simulink model "UR3e_collisional_model"  (R2023b)
settings: Solver=VariableStepAuto  StartTime=0.0  StopTime=60  RelTol=1e-3
model workspace: external: MATLAB File C:\Users\adoma\OneDrive - The University of Manchester\Notes\2023-24\Sem2\Individual Project\Simulation\UR3e\UR3e_DataFile.m (data not in the file)
undefined symbols (not defined in the file): simulation_parameters, smiData, X, Y, Z
libraries: sm_lib x77, nesl_utility x49, robotcorelib x1, robotmaniplib x1
(part 1 of 2)
settings Model: SimulationMode=accelerator  Creator=adoma  LastModifiedBy=user
settings ExplorerConfigSet: SimMechanicsOpenEditorOnUpdate=off

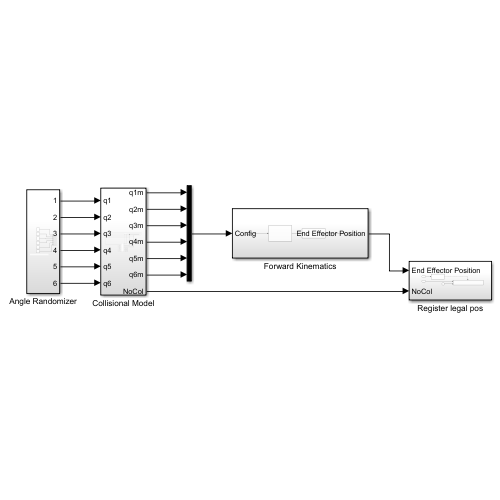
[thumbnail: Simulink's stored preview of the top-level diagram]
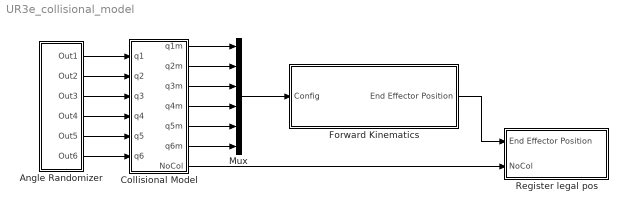
== system UR3e_collisional_model ==
  Angle Randomizer : Subsystem
  Collisional Model : Subsystem
  Forward Kinematics : Subsystem
  Mux : Mux  Inputs=6
  Register legal pos : Subsystem
  wires:
  Mux/1 -> Forward Kinematics/1(Config)
  Collisional Model/1(q1m) -> Mux/1
  Collisional Model/2(q2m) -> Mux/2
  Collisional Model/3(q3m) -> Mux/3
  Collisional Model/4(q4m) -> Mux/4
  Collisional Model/5(q5m) -> Mux/5
  Collisional Model/6(q6m) -> Mux/6
  Forward Kinematics/1(End Effector Position) -> Register legal pos/1(End Effector Position)
  Collisional Model/7(NoCol) -> Register legal pos/2(NoCol)
  Angle Randomizer/1(Out1) -> Collisional Model/1(q1)
  Angle Randomizer/2(Out2) -> Collisional Model/2(q2)
  Angle Randomizer/3(Out3) -> Collisional Model/3(q3)
  Angle Randomizer/4(Out4) -> Collisional Model/4(q4)
  Angle Randomizer/5(Out5) -> Collisional Model/5(q5)
  Angle Randomizer/6(Out6) -> Collisional Model/6(q6)

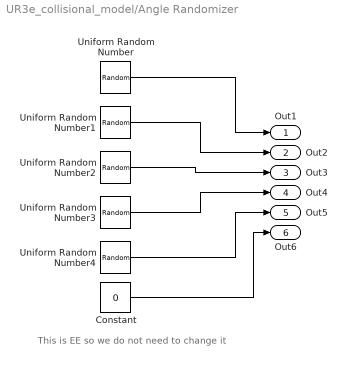
== system UR3e_collisional_model/Angle Randomizer ==
  note: This is EE so we do not need to change it
  Constant : Constant  Value=0
  Uniform Random Number : UniformRandomNumber  Minimum=-pi  Maximum=pi  SampleTime=simulation_parameters.sample_time
  Uniform Random Number1 : UniformRandomNumber  Minimum=-pi  Maximum=pi  Seed=1  SampleTime=simulation_parameters.sample_time
  Uniform Random Number2 : UniformRandomNumber  Minimum=-pi  Maximum=pi  Seed=2  SampleTime=simulation_parameters.sample_time
  Uniform Random Number3 : UniformRandomNumber  Minimum=-pi  Maximum=pi  Seed=3  SampleTime=simulation_parameters.sample_time
  Uniform Random Number4 : UniformRandomNumber  Minimum=-pi  Maximum=pi  Seed=4  SampleTime=simulation_parameters.sample_time
  Out1 : Outport
  Out2 : Outport  Port=2
  Out3 : Outport  Port=3
  Out4 : Outport  Port=4
  Out5 : Outport  Port=5
  Out6 : Outport  Port=6
  wires:
  Uniform Random Number3/1 -> Out4/1
  Uniform Random Number/1 -> Out1/1
  Uniform Random Number1/1 -> Out2/1
  Constant/1 -> Out6/1
  Uniform Random Number4/1 -> Out5/1
  Uniform Random Number2/1 -> Out3/1

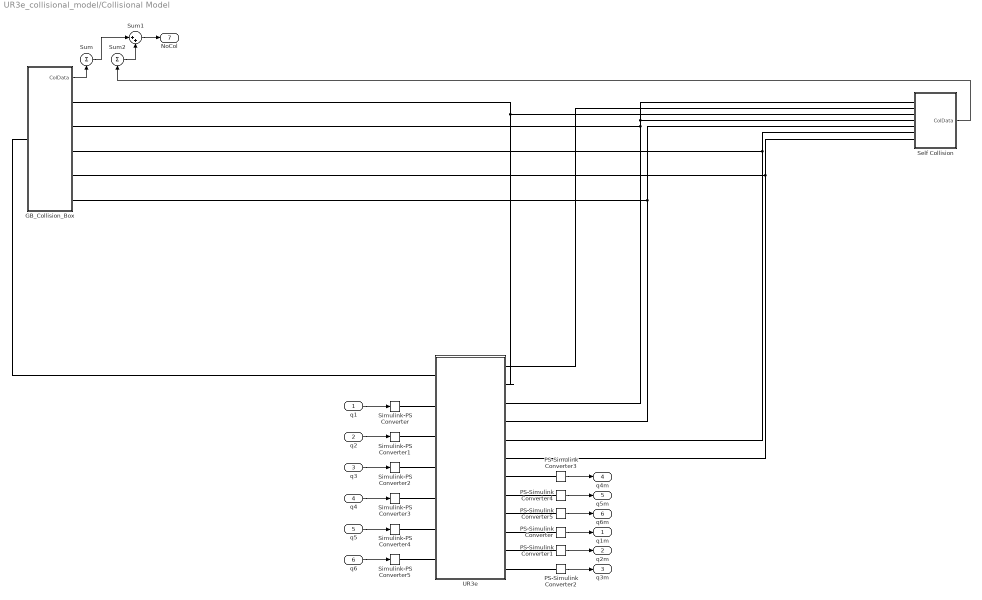
== system UR3e_collisional_model/Collisional Model ==
  q1 : Inport
  q2 : Inport  Port=2
  q3 : Inport  Port=3
  q4 : Inport  Port=4
  q5 : Inport  Port=5
  q6 : Inport  Port=6
  GB_Collision_Box : Subsystem
  PS-Simulink Converter{,1..5} (6 alike) : nesl_utility/PS-Simulink Converter  PhysicalDomain=network_engine_domain  SubClassName=ps_output  LeftPortType=input  RightPortType=output  PseudoPeriodic=off  Frequencies=[]  VectorFormat=inherit  Unit=inherit  AffineConversion=off
  Self Collision : Subsystem
  Simulink-PS Converter{,1..5} (6 alike) : nesl_utility/Simulink-PS Converter  PhysicalDomain=network_engine_domain  SubClassName=ps_input  LeftPortType=input  RightPortType=output  PseudoPeriodic=off  Frequencies=[]  NoiseDistribution=none  NoiseParameters=[]  Unit=rad  AffineConversion=off  FilteringAndDerivatives=filter  SimscapeFilterOrder=2  InputFilterTimeConstant=0.001  UdotUserProvided=0
  Sum : Sum  Inputs=|+
  Sum1 : Sum  Inputs=|++
  Sum2 : Sum  Inputs=|+
  UR3e : Subsystem
  q1m : Outport
  q2m : Outport  Port=2
  q3m : Outport  Port=3
  q4m : Outport  Port=4
  q5m : Outport  Port=5
  q6m : Outport  Port=6
  NoCol : Outport  Port=7
  wires:
  q4/1 -> Simulink-PS Converter3/1
  PS-Simulink Converter3/1 -> q4m/1
  q2/1 -> Simulink-PS Converter1/1
  PS-Simulink Converter1/1 -> q2m/1
  q5/1 -> Simulink-PS Converter4/1
  q3/1 -> Simulink-PS Converter2/1
  PS-Simulink Converter4/1 -> q5m/1
  PS-Simulink Converter5/1 -> q6m/1
  PS-Simulink Converter2/1 -> q3m/1
  q1/1 -> Simulink-PS Converter/1
  PS-Simulink Converter/1 -> q1m/1
  q6/1 -> Simulink-PS Converter5/1
  GB_Collision_Box/1(ColData) -> Sum/1
  Sum/1 -> Sum1/1
  Sum2/1 -> Sum1/2
  Sum1/1 -> NoCol/1
  Self Collision/1(ColData) -> Sum2/1
  connections:
  Self Collision/LConn7 -- UR3e/RConn6 -- GB_Collision_Box/RConn4
  GB_Collision_Box/RConn3 -- UR3e/RConn5 -- Self Collision/LConn6
  GB_Collision_Box/RConn5 -- Self Collision/LConn5 -- UR3e/RConn4
  GB_Collision_Box/LConn1 -- UR3e/LConn1
  Simulink-PS Converter/RConn1 -- UR3e/LConn2
  PS-Simulink Converter3/LConn1 -- UR3e/RConn7
  Simulink-PS Converter1/RConn1 -- UR3e/LConn3
  PS-Simulink Converter4/LConn1 -- UR3e/RConn8
  Simulink-PS Converter2/RConn1 -- UR3e/LConn4
  PS-Simulink Converter5/LConn1 -- UR3e/RConn9
  Simulink-PS Converter3/RConn1 -- UR3e/LConn5
  PS-Simulink Converter/LConn1 -- UR3e/RConn10
  Simulink-PS Converter4/RConn1 -- UR3e/LConn6
  PS-Simulink Converter1/LConn1 -- UR3e/RConn11
  Simulink-PS Converter5/RConn1 -- UR3e/LConn7
  PS-Simulink Converter2/LConn1 -- UR3e/RConn12
  UR3e/RConn2 -- GB_Collision_Box/RConn1 -- Self Collision/LConn3
  GB_Collision_Box/RConn2 -- Self Collision/LConn1 -- Self Collision/LConn4 -- UR3e/RConn3
  UR3e/RConn1 -- Self Collision/LConn2

== system UR3e_collisional_model/Forward Kinematics ==
  Config : Inport
  Coordinate Transformation Conversion : robotcorelib/Coordinate Transformation Conversion  InputRepresentation=Homogeneous Transformation  InputEulerSequence=ZYX  ShowTrVecInputPort=on  OutputRepresentation=Translation Vector  OutputEulerSequence=ZYX  ShowTrVecOutputPort=on  SimulateUsing=Interpreted execution
  Get Transform : robotmaniplib/Get Transform  RigidBodyTree=DOF6_UR3e  SourceBody=Body6  TargetBody=Base  SimulateUsing=Interpreted execution
  End Effector Position : Outport
  wires:
  Get Transform/1 -> Coordinate Transformation Conversion/1
  Coordinate Transformation Conversion/1 -> End Effector Position/1  "End Effector Position"
  Config/1 -> Get Transform/1

== system UR3e_collisional_model/Register legal pos ==
  End Effector Position : Inport
  NoCol : Inport  Port=2
  Clock : Clock
  If : If  IfExpression=u1 == 0  ShowElse=off
  Legal Position Registration : Subsystem  TreatAsAtomicUnit=on
  wires:
  NoCol/1 -> If/1
  If/1 -> Legal Position Registration/Action
  End Effector Position/1 -> Legal Position Registration/1(EE_Pos)
  Clock/1 -> Legal Position Registration/2(SimTime)

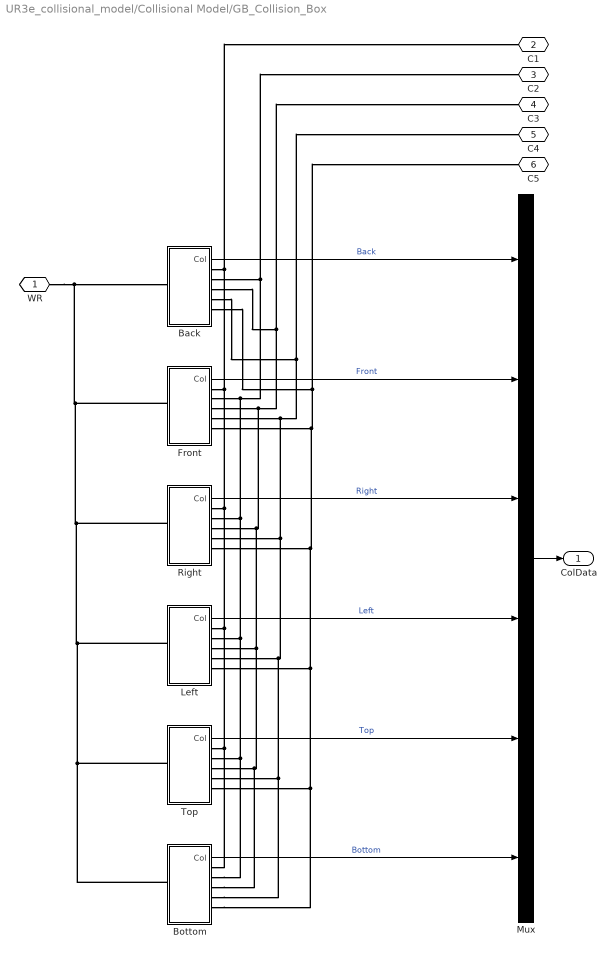
== system UR3e_collisional_model/Collisional Model/GB_Collision_Box ==
  Back : Subsystem
      settings: PortSchema="{\"entries\":[{\"content\":{\"sides\":[{\"content\":{\"connectorIds\":[\"Out1\",\"LConn1\",\"LConn2\",\"LConn3\",\"LConn4\",\"LConn5\"]},\"type\":\"ConnectorPlacement.EquallySpacedRectSide\",\"uuid\":\"f6bf8309-3a61-479f-a747-1123ec87f5cc\"},{\"content\":{\"connectorIds\":[\"RConn1\"],\"side\":\"RIGHT\"},\"type\":\"ConnectorPlacement.EquallySpacedRectSide\",\"uuid\":\"b0f1017d-061c-4274-8acc-6a947b17e7e9\"},{\"content\":{\"side\":\"TOP\"},\"type\":\"ConnectorPlacement.EquallySpacedRectSide\",\"uuid\":\"1775a24a-bc05-4d58-b171-468615c5c014\"}]},\"type\":\"ConnectorPlacement.EquallySpacedConnector\",\"uuid\":\"b2f2d87e-558d-45f7-ad7b-dc693adba59c\"}],\"packageUris\":[\"http://schema.mathworks.com/mf0/Connector/R2020b\"],\"version\":\"1.0\"}"
  Bottom : Subsystem
      settings: PortSchema="{\"entries\":[{\"content\":{\"sides\":[{\"content\":{\"connectorIds\":[\"Out1\",\"LConn1\",\"LConn2\",\"LConn3\",\"LConn4\",\"LConn5\"]},\"type\":\"ConnectorPlacement.EquallySpacedRectSide\",\"uuid\":\"f6bf8309-3a61-479f-a747-1123ec87f5cc\"},{\"content\":{\"connectorIds\":[\"RConn1\"],\"side\":\"RIGHT\"},\"type\":\"ConnectorPlacement.EquallySpacedRectSide\",\"uuid\":\"b0f1017d-061c-4274-8acc-6a947b17e7e9\"},{\"content\":{\"side\":\"TOP\"},\"type\":\"ConnectorPlacement.EquallySpacedRectSide\",\"uuid\":\"1775a24a-bc05-4d58-b171-468615c5c014\"}]},\"type\":\"ConnectorPlacement.EquallySpacedConnector\",\"uuid\":\"b2f2d87e-558d-45f7-ad7b-dc693adba59c\"}],\"packageUris\":[\"http://schema.mathworks.com/mf0/Connector/R2020b\"],\"version\":\"1.0\"}"
  Front : Subsystem
      settings: PortSchema="{\"entries\":[{\"content\":{\"sides\":[{\"content\":{\"connectorIds\":[\"Out1\",\"LConn1\",\"LConn2\",\"LConn3\",\"LConn4\",\"LConn5\"]},\"type\":\"ConnectorPlacement.EquallySpacedRectSide\",\"uuid\":\"f6bf8309-3a61-479f-a747-1123ec87f5cc\"},{\"content\":{\"connectorIds\":[\"RConn1\"],\"side\":\"RIGHT\"},\"type\":\"ConnectorPlacement.EquallySpacedRectSide\",\"uuid\":\"b0f1017d-061c-4274-8acc-6a947b17e7e9\"},{\"content\":{\"side\":\"TOP\"},\"type\":\"ConnectorPlacement.EquallySpacedRectSide\",\"uuid\":\"1775a24a-bc05-4d58-b171-468615c5c014\"}]},\"type\":\"ConnectorPlacement.EquallySpacedConnector\",\"uuid\":\"b2f2d87e-558d-45f7-ad7b-dc693adba59c\"}],\"packageUris\":[\"http://schema.mathworks.com/mf0/Connector/R2020b\"],\"version\":\"1.0\"}"
  Left : Subsystem
      settings: PortSchema="{\"entries\":[{\"content\":{\"sides\":[{\"content\":{\"connectorIds\":[\"Out1\",\"LConn1\",\"LConn2\",\"LConn3\",\"LConn4\",\"LConn5\"]},\"type\":\"ConnectorPlacement.EquallySpacedRectSide\",\"uuid\":\"f6bf8309-3a61-479f-a747-1123ec87f5cc\"},{\"content\":{\"connectorIds\":[\"RConn1\"],\"side\":\"RIGHT\"},\"type\":\"ConnectorPlacement.EquallySpacedRectSide\",\"uuid\":\"b0f1017d-061c-4274-8acc-6a947b17e7e9\"},{\"content\":{\"side\":\"TOP\"},\"type\":\"ConnectorPlacement.EquallySpacedRectSide\",\"uuid\":\"1775a24a-bc05-4d58-b171-468615c5c014\"}]},\"type\":\"ConnectorPlacement.EquallySpacedConnector\",\"uuid\":\"b2f2d87e-558d-45f7-ad7b-dc693adba59c\"}],\"packageUris\":[\"http://schema.mathworks.com/mf0/Connector/R2020b\"],\"version\":\"1.0\"}"
  Mux : Mux  Inputs=6
  Right : Subsystem
      settings: PortSchema="{\"entries\":[{\"content\":{\"sides\":[{\"content\":{\"connectorIds\":[\"Out1\",\"LConn1\",\"LConn2\",\"LConn3\",\"LConn4\",\"LConn5\"]},\"type\":\"ConnectorPlacement.EquallySpacedRectSide\",\"uuid\":\"f6bf8309-3a61-479f-a747-1123ec87f5cc\"},{\"content\":{\"connectorIds\":[\"RConn1\"],\"side\":\"RIGHT\"},\"type\":\"ConnectorPlacement.EquallySpacedRectSide\",\"uuid\":\"b0f1017d-061c-4274-8acc-6a947b17e7e9\"},{\"content\":{\"side\":\"TOP\"},\"type\":\"ConnectorPlacement.EquallySpacedRectSide\",\"uuid\":\"1775a24a-bc05-4d58-b171-468615c5c014\"}]},\"type\":\"ConnectorPlacement.EquallySpacedConnector\",\"uuid\":\"b2f2d87e-558d-45f7-ad7b-dc693adba59c\"}],\"packageUris\":[\"http://schema.mathworks.com/mf0/Connector/R2020b\"],\"version\":\"1.0\"}"
  Top : Subsystem
      settings: PortSchema="{\"entries\":[{\"content\":{\"sides\":[{\"content\":{\"connectorIds\":[\"Out1\",\"LConn1\",\"LConn2\",\"LConn3\",\"LConn4\",\"LConn5\"]},\"type\":\"ConnectorPlacement.EquallySpacedRectSide\",\"uuid\":\"f6bf8309-3a61-479f-a747-1123ec87f5cc\"},{\"content\":{\"connectorIds\":[\"RConn1\"],\"side\":\"RIGHT\"},\"type\":\"ConnectorPlacement.EquallySpacedRectSide\",\"uuid\":\"b0f1017d-061c-4274-8acc-6a947b17e7e9\"},{\"content\":{\"side\":\"TOP\"},\"type\":\"ConnectorPlacement.EquallySpacedRectSide\",\"uuid\":\"1775a24a-bc05-4d58-b171-468615c5c014\"}]},\"type\":\"ConnectorPlacement.EquallySpacedConnector\",\"uuid\":\"b2f2d87e-558d-45f7-ad7b-dc693adba59c\"}],\"packageUris\":[\"http://schema.mathworks.com/mf0/Connector/R2020b\"],\"version\":\"1.0\"}"
  WR : PMIOPort  Side=Left
  C1 : PMIOPort  Port=2  Side=Right
  C2 : PMIOPort  Port=3  Side=Right
  C3 : PMIOPort  Port=4  Side=Right
  C4 : PMIOPort  Port=5  Side=Right
  C5 : PMIOPort  Port=6  Side=Right
  ColData : Outport
  wires:
  Top/1(Col) -> Mux/5  "Top"
  Front/1(Col) -> Mux/2  "Front"
  Bottom/1(Col) -> Mux/6  "Bottom"
  Left/1(Col) -> Mux/4  "Left"
  Back/1(Col) -> Mux/1  "Back"
  Right/1(Col) -> Mux/3  "Right"
  Mux/1 -> ColData/1
  connections:
  Back/LConn4 -- Bottom/LConn4 -- Top/LConn4 -- Left/LConn4 -- Right/LConn4 -- Front/LConn4 -- C4/RConn1
  Back/LConn3 -- Bottom/LConn3 -- Top/LConn3 -- Left/LConn3 -- Right/LConn3 -- Front/LConn3 -- C3/RConn1
  Back/LConn5 -- Bottom/LConn5 -- Top/LConn5 -- Left/LConn5 -- Right/LConn5 -- Front/LConn5 -- C5/RConn1
  Back/LConn1 -- Bottom/LConn1 -- Top/LConn1 -- Left/LConn1 -- Right/LConn1 -- Front/LConn1 -- C1/RConn1
  Back/LConn2 -- Bottom/LConn2 -- Top/LConn2 -- Left/LConn2 -- Right/LConn2 -- Front/LConn2 -- C2/RConn1
  WR/RConn1 -- Bottom/RConn1 -- Top/RConn1 -- Left/RConn1 -- Right/RConn1 -- Front/RConn1 -- Back/RConn1

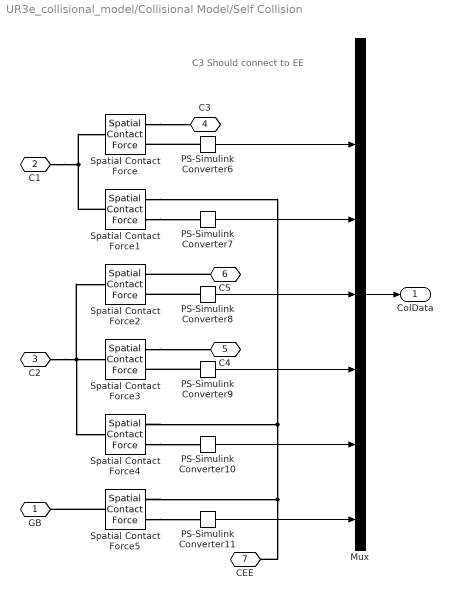
== system UR3e_collisional_model/Collisional Model/Self Collision ==
  note: C3 Should connect to EE
  Mux : Mux  Inputs=7
  PS-Simulink Converter{6..11} (6 alike) : nesl_utility/PS-Simulink Converter  PhysicalDomain=network_engine_domain  SubClassName=ps_output  LeftPortType=input  RightPortType=output  PseudoPeriodic=off  Frequencies=[]  VectorFormat=inherit  Unit=inherit  AffineConversion=off
  Spatial Contact Force{,1,3..5} (5 alike) : sm_lib/Forces and Torques/Spatial Contact Force  SenseContactBaseRotation=off  SenseContactBaseTranslation=off  CoefficientOfDynamicFriction=0.3  CoefficientOfStaticFriction=0.5  NormalDamping=1e3  NormalDampingUnits=N/(m/s)  SenseContactSignal=on  NormalStiffness=1e6  NormalStiffnessUnits=N/m  FrictionalCriticalVelocity=1e-3  FrictionalCriticalVelocityUnits=m/s  ZeroCrossDetectContactStartAndEnd=off  SenseContactFollowerRotation=off  SenseContactFollowerTranslation=off  FrictionType=SmoothStickSlip  SenseFrictionalForceMagnitude=off  SenseNormalForceMagnitude=off  NormalForceType=SmoothSpringDamper  SenseNormalVelocity=off  SensePenetrationDepth=off  SenseSeparationDistance=off  SenseTangentialVelocity=off  NormalTransitionRegionWidth=1e-4  NormalTransitionRegionWidthUnits=m
  Spatial Contact Force2 : sm_lib/Forces and Torques/Spatial Contact Force  SenseContactBaseRotation=off  SenseContactBaseTranslation=off  CoefficientOfDynamicFriction=0.3  CoefficientOfStaticFriction=0.5  NormalDamping=1e3  NormalDampingUnits=N/(m/s)  SenseContactSignal=on  NormalStiffness=1e6  NormalStiffnessUnits=N/m  FrictionalCriticalVelocity=1e-3  FrictionalCriticalVelocityUnits=m/s  ZeroCrossDetectContactStartAndEnd=on  SenseContactFollowerRotation=off  SenseContactFollowerTranslation=off  FrictionType=SmoothStickSlip  SenseFrictionalForceMagnitude=off  SenseNormalForceMagnitude=off  NormalForceType=SmoothSpringDamper  SenseNormalVelocity=off  SensePenetrationDepth=off  SenseSeparationDistance=off  SenseTangentialVelocity=off  NormalTransitionRegionWidth=1e-4  NormalTransitionRegionWidthUnits=m
  GB : PMIOPort  Side=Left
  C1 : PMIOPort  Port=2  Side=Left
  C2 : PMIOPort  Port=3  Side=Left
  C3 : PMIOPort  Port=4  Side=Left
  C4 : PMIOPort  Port=5  Side=Left
  C5 : PMIOPort  Port=6  Side=Left
  CEE : PMIOPort  Port=7  Side=Left
  ColData : Outport
  wires:
  PS-Simulink Converter10/1 -> Mux/6
  PS-Simulink Converter9/1 -> Mux/5
  PS-Simulink Converter8/1 -> Mux/4
  PS-Simulink Converter6/1 -> Mux/2
  PS-Simulink Converter7/1 -> Mux/3
  PS-Simulink Converter11/1 -> Mux/7
  Mux/1 -> ColData/1
  connections:
  C2/RConn1 -- Spatial Contact Force4/LConn1 -- Spatial Contact Force3/LConn1 -- Spatial Contact Force2/LConn1
  Spatial Contact Force3/RConn1 -- C4/RConn1
  PS-Simulink Converter6/LConn1 -- Spatial Contact Force/RConn2
  PS-Simulink Converter8/LConn1 -- Spatial Contact Force2/RConn2
  Spatial Contact Force5/RConn2 -- PS-Simulink Converter11/LConn1
  Spatial Contact Force1/RConn2 -- PS-Simulink Converter7/LConn1
  Spatial Contact Force4/RConn2 -- PS-Simulink Converter10/LConn1
  PS-Simulink Converter9/LConn1 -- Spatial Contact Force3/RConn2
  Spatial Contact Force4/RConn1 -- Spatial Contact Force1/RConn1 -- Spatial Contact Force5/RConn1 -- CEE/RConn1
  Spatial Contact Force5/LConn1 -- GB/RConn1
  C5/RConn1 -- Spatial Contact Force2/RConn1
  C1/RConn1 -- Spatial Contact Force1/LConn1 -- Spatial Contact Force/LConn1
  Spatial Contact Force/RConn1 -- C3/RConn1

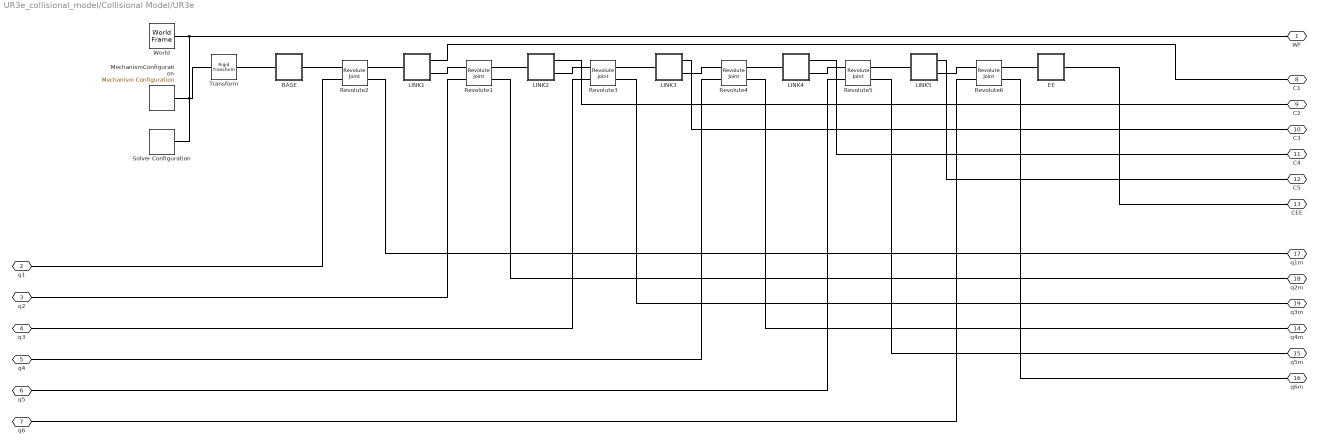
== system UR3e_collisional_model/Collisional Model/UR3e ==
  BASE : Subsystem
  EE : Subsystem
  LINK1 : Subsystem
  LINK2 : Subsystem
  LINK3 : Subsystem
  LINK4 : Subsystem
  LINK5 : Subsystem
  MechanismConfiguration : sm_lib/Utilities/Mechanism Configuration  UniformGravity=Constant  GravityVector=[0 -9.80665 0]  GravityVectorUnits=m/s^2  LinearizationDelta=0.001  JointModeTransitionNonlinearIterations=2
  Revolute{1..5} (5 alike) : sm_lib/Joints/Revolute Joint  JointMode=Normal  SenseConstraintForce=off  SenseConstraintForceX=off  SenseConstraintForceY=off  SenseConstraintForceZ=off  SenseConstraintTorque=off  SenseConstraintTorqueX=off  SenseConstraintTorqueY=off  SenseConstraintTorqueZ=off  SenseTotalForce=off  SenseTotalForceX=off  SenseTotalForceY=off  SenseTotalForceZ=off  SenseTotalTorque=off  SenseTotalTorqueX=off  SenseTotalTorqueY=off  SenseTotalTorqueZ=off  CompositeWrenchDir=FollowerOnBase  CompositeWrenchFrame=BaseFrame  EquilibriumPosition=0  EquilibriumPositionUnits=deg  SpringStiffness=0  SpringStiffnessUnits=N*m/deg  DampingCoefficient=0  DampingCoefficientUnits=N*m/(deg/s)  TorqueActuationMode=ComputedTorque  MotionActuationMode=InputMotion  SensePosition=on  SenseVelocity=off  SenseAcceleration=off  SenseTorqueForce=off  SenseLowerLimitTorqueForce=off  SenseUpperLimitTorqueForce=off  LowerLimitSpecify=on  LowerLimitBound=-360  LowerLimitBoundUnits=deg  LowerLimitStiffness=1e4  LowerLimitStiffnessUnits=N*m/deg  LowerLimitDamping=10  LowerLimitDampingUnits=N*m/(deg/s)  LowerLimitTransitionRegionWidth=0.1  LowerLimitTransitionRegionWidthUnits=deg  UpperLimitSpecify=on  UpperLimitBound=360  UpperLimitBoundUnits=deg  UpperLimitStiffness=1e4  UpperLimitStiffnessUnits=N*m/deg  UpperLimitDamping=10  UpperLimitDampingUnits=N*m/(deg/s)  UpperLimitTransitionRegionWidth=0.1  UpperLimitTransitionRegionWidthUnits=deg  PositionTargetSpecify=on  PositionTargetPriority=Low  PositionTargetValue=smiData.RevoluteJoint(3).Rz.Pos  PositionTargetValueUnits=deg  VelocityTargetSpecify=off  VelocityTargetPriority=High  VelocityTargetValue=0  VelocityTargetValueUnits=deg/s
  Revolute6 : sm_lib/Joints/Revolute Joint  JointMode=Normal  SenseConstraintForce=off  SenseConstraintForceX=off  SenseConstraintForceY=off  SenseConstraintForceZ=off  SenseConstraintTorque=off  SenseConstraintTorqueX=off  SenseConstraintTorqueY=off  SenseConstraintTorqueZ=off  SenseTotalForce=off  SenseTotalForceX=off  SenseTotalForceY=off  SenseTotalForceZ=off  SenseTotalTorque=off  SenseTotalTorqueX=off  SenseTotalTorqueY=off  SenseTotalTorqueZ=off  CompositeWrenchDir=FollowerOnBase  CompositeWrenchFrame=BaseFrame  EquilibriumPosition=0  EquilibriumPositionUnits=deg  SpringStiffness=0  SpringStiffnessUnits=N*m/deg  DampingCoefficient=0  DampingCoefficientUnits=N*m/(deg/s)  TorqueActuationMode=ComputedTorque  MotionActuationMode=InputMotion  SensePosition=on  SenseVelocity=off  SenseAcceleration=off  SenseTorqueForce=off  SenseLowerLimitTorqueForce=off  SenseUpperLimitTorqueForce=off  LowerLimitSpecify=off  LowerLimitBound=-360  LowerLimitBoundUnits=deg  LowerLimitStiffness=1e4  LowerLimitStiffnessUnits=N*m/deg  LowerLimitDamping=10  LowerLimitDampingUnits=N*m/(deg/s)  LowerLimitTransitionRegionWidth=0.1  LowerLimitTransitionRegionWidthUnits=deg  UpperLimitSpecify=off  UpperLimitBound=360  UpperLimitBoundUnits=deg  UpperLimitStiffness=1e4  UpperLimitStiffnessUnits=N*m/deg  UpperLimitDamping=10  UpperLimitDampingUnits=N*m/(deg/s)  UpperLimitTransitionRegionWidth=0.1  UpperLimitTransitionRegionWidthUnits=deg  PositionTargetSpecify=on  PositionTargetPriority=Low  PositionTargetValue=smiData.RevoluteJoint(3).Rz.Pos  PositionTargetValueUnits=deg  VelocityTargetSpecify=off  VelocityTargetPriority=High  VelocityTargetValue=0  VelocityTargetValueUnits=deg/s
  Solver Configuration : nesl_utility/Solver Configuration  PhysicalDomain=network_engine_domain  SubClassName=solver  LeftPortType=input  RightPortType=generic  Tones=[]  Harmonics=[]  SimulateNoise=off  Profile=off  UseLocalSampling=off  EnableSwitchedLinearOptims=on  FrequencyDomain=off  UseCCode=off  RelTol=0.001  AbsTol=0.001  MinStep=1e-09  ToWorkspace=off  RevertToSquareIcSolve=off  NumHomotopyIterations=100  PhasorMode=off  PhasorModeNumHarmonics=1  ConsistencySolver=NEWTON_XTOL_AFTER_FTOL  IndexReductionMethod=DerivativeReplacement  DoDC=off  ResidualTolerance=1e-09  ConsistencyTolSource=GLOBAL  ConsistencyAbsTol=0.001  ConsistencyRelTol=0.001  ConsistencyTolFactor=0.001  UseLocalSolver=off  LocalSolverChoice=NE_BACKWARD_EULER_ADVANCER  ResolveIndetEquations=on  FunctionEvalNumThread=1  LocalSolverSampleTime=0.001  DoFixedCost=off  MaxNonlinIter=3  MaxModeIter=2  ComputeImpulses=off  ImpulseIterations=2  LinearAlgebra=auto  LinearAlgebraNumThread=0  EquationFormulation=NE_TIME_EF  DelaysMemoryBudget=1024  AutomaticFiltering=on  FilteringTimeConstant=0.001  PartitionStorageMethod=AS_NEEDED  PartitionMemoryBudget=1024  PartitionMethod=ROBUST  MultibodyUseLocalSolver=off  MultibodyLocalSolverChoice=ODE1  MultibodyLocalSolverSampleTime=0.001
  Transform : sm_lib/Frames and Transforms/Rigid Transform  TranslationMethod=Cartesian  TranslationStandardOffset=0  TranslationStandardOffsetUnits=m  TranslationStandardAxis=+Z  TranslationCartesianOffset=smiData.RigidTransform(13).translation  TranslationCartesianOffsetUnits=mm  TranslationROffset=0  TranslationROffsetUnits=m  TranslationZOffset=0  TranslationZOffsetUnits=m  TranslationThetaOffset=0  TranslationThetaOffsetUnits=deg  RotationMethod=ArbitraryAxis  RotationAngleUnits=rad  RotationStandardAxis=+Z  RotationAngle=smiData.RigidTransform(13).angle  RotationArbitraryAxis=smiData.RigidTransform(13).axis  FollAlignAxisA=+X  BaseAlignAxisA=+Y  FollAlignAxisB=+Y  BaseAlignAxisB=+Z  RotationSequenceAxes=FollowerAxes  RotationSequence=XYX  RotationSequenceAngles=[0 0 0]  RotationSequenceAnglesUnits=deg  RotationMatrix=[1 0 0; 0 1 0; 0 0 1]  Quaternion=[1 0 0 0]
  World : sm_lib/Frames and Transforms/World Frame
  WF : PMIOPort  Side=Left
  q1 : PMIOPort  Port=2  Side=Left
  q2 : PMIOPort  Port=3  Side=Left
  q3 : PMIOPort  Port=4  Side=Left
  q4 : PMIOPort  Port=5  Side=Left
  q5 : PMIOPort  Port=6  Side=Left
  q6 : PMIOPort  Port=7  Side=Left
  C1 : PMIOPort  Port=8  Side=Right
  C2 : PMIOPort  Port=9  Side=Right
  C3 : PMIOPort  Port=10  Side=Right
  C4 : PMIOPort  Port=11  Side=Right
  C5 : PMIOPort  Port=12  Side=Right
  CEE : PMIOPort  Port=13  Side=Right
  q4m : PMIOPort  Port=14  Side=Right
  q5m : PMIOPort  Port=15  Side=Right
  q6m : PMIOPort  Port=16  Side=Right
  q1m : PMIOPort  Port=17  Side=Right
  q2m : PMIOPort  Port=18  Side=Right
  q3m : PMIOPort  Port=19  Side=Right
  connections:
  MechanismConfiguration/RConn1 -- Solver Configuration/RConn1 -- Transform/LConn1 -- WF/RConn1 -- World/RConn1
  Revolute4/LConn1 -- LINK3/RConn2
  Revolute5/LConn1 -- LINK4/RConn2
  Revolute4/RConn1 -- LINK4/LConn1
  Revolute3/RConn1 -- LINK3/LConn1
  LINK1/LConn1 -- Revolute2/RConn1
  Revolute6/RConn1 -- EE/LConn1
  BASE/LConn1 -- Transform/RConn1
  Revolute1/LConn1 -- LINK1/RConn2
  Revolute3/LConn1 -- LINK2/RConn2
  BASE/RConn1 -- Revolute2/LConn1
  Revolute6/LConn1 -- LINK5/RConn2
  Revolute1/RConn1 -- LINK2/LConn1
  Revolute5/RConn1 -- LINK5/LConn1
  q1/RConn1 -- Revolute2/LConn2
  q2/RConn1 -- Revolute1/LConn2
  q3/RConn1 -- Revolute3/LConn2
  q4/RConn1 -- Revolute4/LConn2
  q5/RConn1 -- Revolute5/LConn2
  q6/RConn1 -- Revolute6/LConn2
  Revolute2/RConn2 -- q1m/RConn1
  Revolute1/RConn2 -- q2m/RConn1
  Revolute3/RConn2 -- q3m/RConn1
  Revolute4/RConn2 -- q4m/RConn1
  Revolute5/RConn2 -- q5m/RConn1
  Revolute6/RConn2 -- q6m/RConn1
  LINK1/RConn1 -- C1/RConn1
  LINK2/RConn1 -- C2/RConn1
  LINK3/RConn1 -- C3/RConn1
  LINK4/RConn1 -- C4/RConn1
  LINK5/RConn1 -- C5/RConn1
  EE/RConn1 -- CEE/RConn1

== system UR3e_collisional_model/Register legal pos/Legal Position Registration ==
  EE_Pos : Inport
  SimTime : Inport  Port=2
  Action Port : ActionPort  ActionPortLabel=if(u1 == 0)
  To File : ToFile  Filename=simout.mat  MatrixName=legal_positions
  To File1 : ToFile  Commented=on  Filename=simout.mat  MatrixName=leg_time  SaveFormat=Timeseries
  wires:
  EE_Pos/1 -> To File/1
  SimTime/1 -> To File1/1

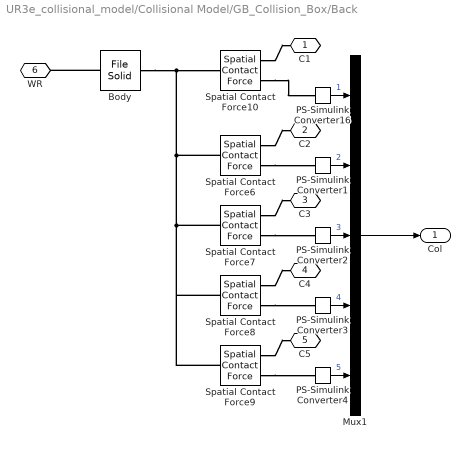
== system UR3e_collisional_model/Collisional Model/GB_Collision_Box/Back ==
  Body : sm_lib/Body Elements/File Solid  ExtGeomFileName=\UR3e_simscape_models\Glovebox_models\Back.stp  UnitType=FromFile  ExtGeomFileUnits=m  StepReaderType=HEX  ExportConvexHullGeometry=on  InertiaType=Custom  Mass=0  MassUnits=kg  CenterOfMass=[0 0 0]  CenterOfMassUnits=m  MomentsOfInertia=[1 1 1]  MomentsOfInertiaUnits=kg*m^2  ProductsOfInertia=[0 0 0]  ProductsOfInertiaUnits=kg*m^2  BasedOnType=DensityFromFile  Density=1000  DensityUnits=kg/m^3  DoExposeReferenceFrame=on  SerializedFrames=<Frames/>  GraphicType=FromGeometry  MarkerShape=Sphere  MarkerSize=10  GraphicVisPropType=SimpleVisualProperties  GraphicDiffuseColor=[1.0 1.0 1.0]  GraphicSpecularColor=[0.5 0.5 0.5 1.0]  GraphicAmbientColor=[0.15 0.15 0.15 1.0]  GraphicEmissiveColor=[0.0 0.0 0.0 1.0]  GraphicShininess=75  GraphicOpacity=0.2
  Mux1 : Mux  Inputs=5
  PS-Simulink Converter{1..4,16} (5 alike) : nesl_utility/PS-Simulink Converter  PhysicalDomain=network_engine_domain  SubClassName=ps_output  LeftPortType=input  RightPortType=output  PseudoPeriodic=off  Frequencies=[]  VectorFormat=inherit  Unit=inherit  AffineConversion=off
  Spatial Contact Force{7..10} (4 alike) : sm_lib/Forces and Torques/Spatial Contact Force  SenseContactBaseRotation=off  SenseContactBaseTranslation=off  CoefficientOfDynamicFriction=0.3  CoefficientOfStaticFriction=0.5  NormalDamping=1e3  NormalDampingUnits=N/(m/s)  SenseContactSignal=on  NormalStiffness=1e6  NormalStiffnessUnits=N/m  FrictionalCriticalVelocity=1e-3  FrictionalCriticalVelocityUnits=m/s  ZeroCrossDetectContactStartAndEnd=off  SenseContactFollowerRotation=off  SenseContactFollowerTranslation=off  FrictionType=SmoothStickSlip  SenseFrictionalForceMagnitude=off  SenseNormalForceMagnitude=off  NormalForceType=SmoothSpringDamper  SenseNormalVelocity=off  SensePenetrationDepth=off  SenseSeparationDistance=off  SenseTangentialVelocity=off  NormalTransitionRegionWidth=1e-4  NormalTransitionRegionWidthUnits=m
  Spatial Contact Force6 : sm_lib/Forces and Torques/Spatial Contact Force  SenseContactBaseRotation=off  SenseContactBaseTranslation=off  CoefficientOfDynamicFriction=0.3  CoefficientOfStaticFriction=0.5  NormalDamping=1e3  NormalDampingUnits=N/(m/s)  SenseContactSignal=on  NormalStiffness=1e6  NormalStiffnessUnits=N/m  FrictionalCriticalVelocity=1e-3  FrictionalCriticalVelocityUnits=m/s  ZeroCrossDetectContactStartAndEnd=on  SenseContactFollowerRotation=off  SenseContactFollowerTranslation=off  FrictionType=SmoothStickSlip  SenseFrictionalForceMagnitude=off  SenseNormalForceMagnitude=off  NormalForceType=SmoothSpringDamper  SenseNormalVelocity=off  SensePenetrationDepth=off  SenseSeparationDistance=off  SenseTangentialVelocity=off  NormalTransitionRegionWidth=1e-4  NormalTransitionRegionWidthUnits=m
  C1 : PMIOPort  Side=Left
  C2 : PMIOPort  Port=2  Side=Left
  C3 : PMIOPort  Port=3  Side=Left
  C4 : PMIOPort  Port=4  Side=Left
  C5 : PMIOPort  Port=5  Side=Left
  WR : PMIOPort  Port=6  Side=Right
  Col : Outport
  wires:
  PS-Simulink Converter4/1 -> Mux1/5  "5"
  PS-Simulink Converter3/1 -> Mux1/4  "4"
  PS-Simulink Converter16/1 -> Mux1/1  "1"
  PS-Simulink Converter1/1 -> Mux1/2  "2"
  PS-Simulink Converter2/1 -> Mux1/3  "3"
  Mux1/1 -> Col/1
  connections:
  Body/RConn1 -- WR/RConn1
  Body/LConn1 -- Spatial Contact Force10/LConn1 -- Spatial Contact Force9/LConn1 -- Spatial Contact Force8/LConn1 -- Spatial Contact Force7/LConn1 -- Spatial Contact Force6/LConn1
  Spatial Contact Force10/RConn1 -- C1/RConn1
  Spatial Contact Force8/RConn2 -- PS-Simulink Converter3/LConn1
  Spatial Contact Force7/RConn2 -- PS-Simulink Converter2/LConn1
  Spatial Contact Force9/RConn2 -- PS-Simulink Converter4/LConn1
  Spatial Contact Force6/RConn2 -- PS-Simulink Converter1/LConn1
  Spatial Contact Force10/RConn2 -- PS-Simulink Converter16/LConn1
  Spatial Contact Force6/RConn1 -- C2/RConn1
  Spatial Contact Force7/RConn1 -- C3/RConn1
  Spatial Contact Force8/RConn1 -- C4/RConn1
  Spatial Contact Force9/RConn1 -- C5/RConn1

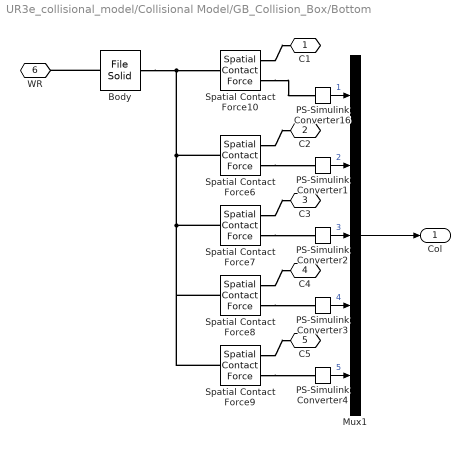
== system UR3e_collisional_model/Collisional Model/GB_Collision_Box/Bottom ==
  Body : sm_lib/Body Elements/File Solid  ExtGeomFileName=\UR3e_simscape_models\Glovebox_models\Bottom.stp  UnitType=FromFile  ExtGeomFileUnits=m  StepReaderType=HEX  ExportConvexHullGeometry=on  InertiaType=Custom  Mass=0  MassUnits=kg  CenterOfMass=[0 0 0]  CenterOfMassUnits=m  MomentsOfInertia=[1 1 1]  MomentsOfInertiaUnits=kg*m^2  ProductsOfInertia=[0 0 0]  ProductsOfInertiaUnits=kg*m^2  BasedOnType=DensityFromFile  Density=1000  DensityUnits=kg/m^3  DoExposeReferenceFrame=on  SerializedFrames=<Frames/>  GraphicType=FromGeometry  MarkerShape=Sphere  MarkerSize=10  GraphicVisPropType=SimpleVisualProperties  GraphicDiffuseColor=[1.0 1.0 1.0]  GraphicSpecularColor=[0.5 0.5 0.5 1.0]  GraphicAmbientColor=[0.15 0.15 0.15 1.0]  GraphicEmissiveColor=[0.0 0.0 0.0 1.0]  GraphicShininess=75  GraphicOpacity=0.2
  Mux1 : Mux  Inputs=5
  PS-Simulink Converter{1..4,16} (5 alike) : nesl_utility/PS-Simulink Converter  PhysicalDomain=network_engine_domain  SubClassName=ps_output  LeftPortType=input  RightPortType=output  PseudoPeriodic=off  Frequencies=[]  VectorFormat=inherit  Unit=inherit  AffineConversion=off
  Spatial Contact Force{7..10} (4 alike) : sm_lib/Forces and Torques/Spatial Contact Force  SenseContactBaseRotation=off  SenseContactBaseTranslation=off  CoefficientOfDynamicFriction=0.3  CoefficientOfStaticFriction=0.5  NormalDamping=1e3  NormalDampingUnits=N/(m/s)  SenseContactSignal=on  NormalStiffness=1e6  NormalStiffnessUnits=N/m  FrictionalCriticalVelocity=1e-3  FrictionalCriticalVelocityUnits=m/s  ZeroCrossDetectContactStartAndEnd=off  SenseContactFollowerRotation=off  SenseContactFollowerTranslation=off  FrictionType=SmoothStickSlip  SenseFrictionalForceMagnitude=off  SenseNormalForceMagnitude=off  NormalForceType=SmoothSpringDamper  SenseNormalVelocity=off  SensePenetrationDepth=off  SenseSeparationDistance=off  SenseTangentialVelocity=off  NormalTransitionRegionWidth=1e-4  NormalTransitionRegionWidthUnits=m
  Spatial Contact Force6 : sm_lib/Forces and Torques/Spatial Contact Force  SenseContactBaseRotation=off  SenseContactBaseTranslation=off  CoefficientOfDynamicFriction=0.3  CoefficientOfStaticFriction=0.5  NormalDamping=1e3  NormalDampingUnits=N/(m/s)  SenseContactSignal=on  NormalStiffness=1e6  NormalStiffnessUnits=N/m  FrictionalCriticalVelocity=1e-3  FrictionalCriticalVelocityUnits=m/s  ZeroCrossDetectContactStartAndEnd=on  SenseContactFollowerRotation=off  SenseContactFollowerTranslation=off  FrictionType=SmoothStickSlip  SenseFrictionalForceMagnitude=off  SenseNormalForceMagnitude=off  NormalForceType=SmoothSpringDamper  SenseNormalVelocity=off  SensePenetrationDepth=off  SenseSeparationDistance=off  SenseTangentialVelocity=off  NormalTransitionRegionWidth=1e-4  NormalTransitionRegionWidthUnits=m
  C1 : PMIOPort  Side=Left
  C2 : PMIOPort  Port=2  Side=Left
  C3 : PMIOPort  Port=3  Side=Left
  C4 : PMIOPort  Port=4  Side=Left
  C5 : PMIOPort  Port=5  Side=Left
  WR : PMIOPort  Port=6  Side=Right
  Col : Outport
  wires:
  PS-Simulink Converter4/1 -> Mux1/5  "5"
  PS-Simulink Converter3/1 -> Mux1/4  "4"
  PS-Simulink Converter16/1 -> Mux1/1  "1"
  PS-Simulink Converter1/1 -> Mux1/2  "2"
  PS-Simulink Converter2/1 -> Mux1/3  "3"
  Mux1/1 -> Col/1
  connections:
  Body/RConn1 -- WR/RConn1
  Body/LConn1 -- Spatial Contact Force9/LConn1 -- Spatial Contact Force8/LConn1 -- Spatial Contact Force7/LConn1 -- Spatial Contact Force6/LConn1 -- Spatial Contact Force10/LConn1
  Spatial Contact Force10/RConn1 -- C1/RConn1
  Spatial Contact Force8/RConn2 -- PS-Simulink Converter3/LConn1
  Spatial Contact Force7/RConn2 -- PS-Simulink Converter2/LConn1
  Spatial Contact Force9/RConn2 -- PS-Simulink Converter4/LConn1
  Spatial Contact Force6/RConn2 -- PS-Simulink Converter1/LConn1
  Spatial Contact Force10/RConn2 -- PS-Simulink Converter16/LConn1
  Spatial Contact Force6/RConn1 -- C2/RConn1
  Spatial Contact Force7/RConn1 -- C3/RConn1
  Spatial Contact Force8/RConn1 -- C4/RConn1
  Spatial Contact Force9/RConn1 -- C5/RConn1

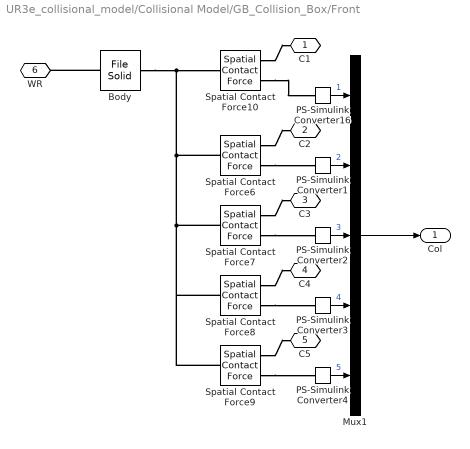
== system UR3e_collisional_model/Collisional Model/GB_Collision_Box/Front ==
  Body : sm_lib/Body Elements/File Solid  ExtGeomFileName=\UR3e_simscape_models\Glovebox_models\Front.stp  UnitType=FromFile  ExtGeomFileUnits=m  StepReaderType=HEX  ExportConvexHullGeometry=on  InertiaType=Custom  Mass=0  MassUnits=kg  CenterOfMass=[0 0 0]  CenterOfMassUnits=m  MomentsOfInertia=[1 1 1]  MomentsOfInertiaUnits=kg*m^2  ProductsOfInertia=[0 0 0]  ProductsOfInertiaUnits=kg*m^2  BasedOnType=DensityFromFile  Density=1000  DensityUnits=kg/m^3  DoExposeReferenceFrame=on  SerializedFrames=<Frames/>  GraphicType=FromGeometry  MarkerShape=Sphere  MarkerSize=10  GraphicVisPropType=SimpleVisualProperties  GraphicDiffuseColor=[1.0 1.0 1.0]  GraphicSpecularColor=[0.5 0.5 0.5 1.0]  GraphicAmbientColor=[0.15 0.15 0.15 1.0]  GraphicEmissiveColor=[0.0 0.0 0.0 1.0]  GraphicShininess=75  GraphicOpacity=0.2
  Mux1 : Mux  Inputs=5
  PS-Simulink Converter{1..4,16} (5 alike) : nesl_utility/PS-Simulink Converter  PhysicalDomain=network_engine_domain  SubClassName=ps_output  LeftPortType=input  RightPortType=output  PseudoPeriodic=off  Frequencies=[]  VectorFormat=inherit  Unit=inherit  AffineConversion=off
  Spatial Contact Force{7..10} (4 alike) : sm_lib/Forces and Torques/Spatial Contact Force  SenseContactBaseRotation=off  SenseContactBaseTranslation=off  CoefficientOfDynamicFriction=0.3  CoefficientOfStaticFriction=0.5  NormalDamping=1e3  NormalDampingUnits=N/(m/s)  SenseContactSignal=on  NormalStiffness=1e6  NormalStiffnessUnits=N/m  FrictionalCriticalVelocity=1e-3  FrictionalCriticalVelocityUnits=m/s  ZeroCrossDetectContactStartAndEnd=off  SenseContactFollowerRotation=off  SenseContactFollowerTranslation=off  FrictionType=SmoothStickSlip  SenseFrictionalForceMagnitude=off  SenseNormalForceMagnitude=off  NormalForceType=SmoothSpringDamper  SenseNormalVelocity=off  SensePenetrationDepth=off  SenseSeparationDistance=off  SenseTangentialVelocity=off  NormalTransitionRegionWidth=1e-4  NormalTransitionRegionWidthUnits=m
  Spatial Contact Force6 : sm_lib/Forces and Torques/Spatial Contact Force  SenseContactBaseRotation=off  SenseContactBaseTranslation=off  CoefficientOfDynamicFriction=0.3  CoefficientOfStaticFriction=0.5  NormalDamping=1e3  NormalDampingUnits=N/(m/s)  SenseContactSignal=on  NormalStiffness=1e6  NormalStiffnessUnits=N/m  FrictionalCriticalVelocity=1e-3  FrictionalCriticalVelocityUnits=m/s  ZeroCrossDetectContactStartAndEnd=on  SenseContactFollowerRotation=off  SenseContactFollowerTranslation=off  FrictionType=SmoothStickSlip  SenseFrictionalForceMagnitude=off  SenseNormalForceMagnitude=off  NormalForceType=SmoothSpringDamper  SenseNormalVelocity=off  SensePenetrationDepth=off  SenseSeparationDistance=off  SenseTangentialVelocity=off  NormalTransitionRegionWidth=1e-4  NormalTransitionRegionWidthUnits=m
  C1 : PMIOPort  Side=Left
  C2 : PMIOPort  Port=2  Side=Left
  C3 : PMIOPort  Port=3  Side=Left
  C4 : PMIOPort  Port=4  Side=Left
  C5 : PMIOPort  Port=5  Side=Left
  WR : PMIOPort  Port=6  Side=Right
  Col : Outport
  wires:
  PS-Simulink Converter4/1 -> Mux1/5  "5"
  PS-Simulink Converter3/1 -> Mux1/4  "4"
  PS-Simulink Converter16/1 -> Mux1/1  "1"
  PS-Simulink Converter1/1 -> Mux1/2  "2"
  PS-Simulink Converter2/1 -> Mux1/3  "3"
  Mux1/1 -> Col/1
  connections:
  Body/RConn1 -- WR/RConn1
  Body/LConn1 -- Spatial Contact Force10/LConn1 -- Spatial Contact Force9/LConn1 -- Spatial Contact Force8/LConn1 -- Spatial Contact Force7/LConn1 -- Spatial Contact Force6/LConn1
  Spatial Contact Force10/RConn1 -- C1/RConn1
  Spatial Contact Force8/RConn2 -- PS-Simulink Converter3/LConn1
  Spatial Contact Force7/RConn2 -- PS-Simulink Converter2/LConn1
  Spatial Contact Force9/RConn2 -- PS-Simulink Converter4/LConn1
  Spatial Contact Force6/RConn2 -- PS-Simulink Converter1/LConn1
  Spatial Contact Force10/RConn2 -- PS-Simulink Converter16/LConn1
  Spatial Contact Force6/RConn1 -- C2/RConn1
  Spatial Contact Force7/RConn1 -- C3/RConn1
  Spatial Contact Force8/RConn1 -- C4/RConn1
  Spatial Contact Force9/RConn1 -- C5/RConn1

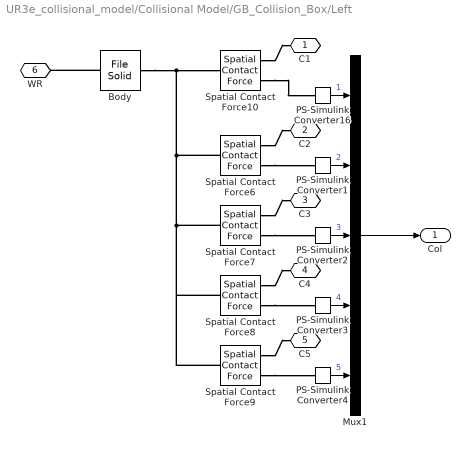
== system UR3e_collisional_model/Collisional Model/GB_Collision_Box/Left ==
  Body : sm_lib/Body Elements/File Solid  ExtGeomFileName=\UR3e_simscape_models\Glovebox_models\Left.stp  UnitType=FromFile  ExtGeomFileUnits=m  StepReaderType=HEX  ExportConvexHullGeometry=on  InertiaType=Custom  Mass=0  MassUnits=kg  CenterOfMass=[0 0 0]  CenterOfMassUnits=m  MomentsOfInertia=[1 1 1]  MomentsOfInertiaUnits=kg*m^2  ProductsOfInertia=[0 0 0]  ProductsOfInertiaUnits=kg*m^2  BasedOnType=DensityFromFile  Density=1000  DensityUnits=kg/m^3  DoExposeReferenceFrame=on  SerializedFrames=<Frames/>  GraphicType=FromGeometry  MarkerShape=Sphere  MarkerSize=10  GraphicVisPropType=SimpleVisualProperties  GraphicDiffuseColor=[1.0 1.0 1.0]  GraphicSpecularColor=[0.5 0.5 0.5 1.0]  GraphicAmbientColor=[0.15 0.15 0.15 1.0]  GraphicEmissiveColor=[0.0 0.0 0.0 1.0]  GraphicShininess=75  GraphicOpacity=0.2
  Mux1 : Mux  Inputs=5
  PS-Simulink Converter{1..4,16} (5 alike) : nesl_utility/PS-Simulink Converter  PhysicalDomain=network_engine_domain  SubClassName=ps_output  LeftPortType=input  RightPortType=output  PseudoPeriodic=off  Frequencies=[]  VectorFormat=inherit  Unit=inherit  AffineConversion=off
  Spatial Contact Force{7..10} (4 alike) : sm_lib/Forces and Torques/Spatial Contact Force  SenseContactBaseRotation=off  SenseContactBaseTranslation=off  CoefficientOfDynamicFriction=0.3  CoefficientOfStaticFriction=0.5  NormalDamping=1e3  NormalDampingUnits=N/(m/s)  SenseContactSignal=on  NormalStiffness=1e6  NormalStiffnessUnits=N/m  FrictionalCriticalVelocity=1e-3  FrictionalCriticalVelocityUnits=m/s  ZeroCrossDetectContactStartAndEnd=off  SenseContactFollowerRotation=off  SenseContactFollowerTranslation=off  FrictionType=SmoothStickSlip  SenseFrictionalForceMagnitude=off  SenseNormalForceMagnitude=off  NormalForceType=SmoothSpringDamper  SenseNormalVelocity=off  SensePenetrationDepth=off  SenseSeparationDistance=off  SenseTangentialVelocity=off  NormalTransitionRegionWidth=1e-4  NormalTransitionRegionWidthUnits=m
  Spatial Contact Force6 : sm_lib/Forces and Torques/Spatial Contact Force  SenseContactBaseRotation=off  SenseContactBaseTranslation=off  CoefficientOfDynamicFriction=0.3  CoefficientOfStaticFriction=0.5  NormalDamping=1e3  NormalDampingUnits=N/(m/s)  SenseContactSignal=on  NormalStiffness=1e6  NormalStiffnessUnits=N/m  FrictionalCriticalVelocity=1e-3  FrictionalCriticalVelocityUnits=m/s  ZeroCrossDetectContactStartAndEnd=on  SenseContactFollowerRotation=off  SenseContactFollowerTranslation=off  FrictionType=SmoothStickSlip  SenseFrictionalForceMagnitude=off  SenseNormalForceMagnitude=off  NormalForceType=SmoothSpringDamper  SenseNormalVelocity=off  SensePenetrationDepth=off  SenseSeparationDistance=off  SenseTangentialVelocity=off  NormalTransitionRegionWidth=1e-4  NormalTransitionRegionWidthUnits=m
  C1 : PMIOPort  Side=Left
  C2 : PMIOPort  Port=2  Side=Left
  C3 : PMIOPort  Port=3  Side=Left
  C4 : PMIOPort  Port=4  Side=Left
  C5 : PMIOPort  Port=5  Side=Left
  WR : PMIOPort  Port=6  Side=Right
  Col : Outport
  wires:
  PS-Simulink Converter4/1 -> Mux1/5  "5"
  PS-Simulink Converter3/1 -> Mux1/4  "4"
  PS-Simulink Converter16/1 -> Mux1/1  "1"
  PS-Simulink Converter1/1 -> Mux1/2  "2"
  PS-Simulink Converter2/1 -> Mux1/3  "3"
  Mux1/1 -> Col/1
  connections:
  Body/RConn1 -- WR/RConn1
  Body/LConn1 -- Spatial Contact Force10/LConn1 -- Spatial Contact Force9/LConn1 -- Spatial Contact Force8/LConn1 -- Spatial Contact Force7/LConn1 -- Spatial Contact Force6/LConn1
  Spatial Contact Force10/RConn1 -- C1/RConn1
  Spatial Contact Force8/RConn2 -- PS-Simulink Converter3/LConn1
  Spatial Contact Force7/RConn2 -- PS-Simulink Converter2/LConn1
  Spatial Contact Force9/RConn2 -- PS-Simulink Converter4/LConn1
  Spatial Contact Force6/RConn2 -- PS-Simulink Converter1/LConn1
  Spatial Contact Force10/RConn2 -- PS-Simulink Converter16/LConn1
  Spatial Contact Force6/RConn1 -- C2/RConn1
  Spatial Contact Force7/RConn1 -- C3/RConn1
  Spatial Contact Force8/RConn1 -- C4/RConn1
  Spatial Contact Force9/RConn1 -- C5/RConn1

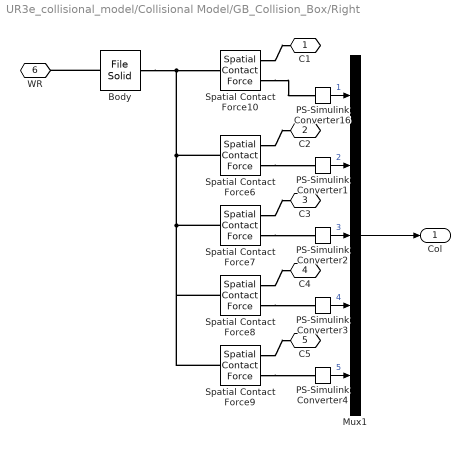
== system UR3e_collisional_model/Collisional Model/GB_Collision_Box/Right ==
  Body : sm_lib/Body Elements/File Solid  ExtGeomFileName=\UR3e_simscape_models\Glovebox_models\Right.stp  UnitType=FromFile  ExtGeomFileUnits=m  StepReaderType=HEX  ExportConvexHullGeometry=on  InertiaType=Custom  Mass=0  MassUnits=kg  CenterOfMass=[0 0 0]  CenterOfMassUnits=m  MomentsOfInertia=[1 1 1]  MomentsOfInertiaUnits=kg*m^2  ProductsOfInertia=[0 0 0]  ProductsOfInertiaUnits=kg*m^2  BasedOnType=DensityFromFile  Density=1000  DensityUnits=kg/m^3  DoExposeReferenceFrame=on  SerializedFrames=<Frames/>  GraphicType=FromGeometry  MarkerShape=Sphere  MarkerSize=10  GraphicVisPropType=SimpleVisualProperties  GraphicDiffuseColor=[1.0 1.0 1.0]  GraphicSpecularColor=[0.5 0.5 0.5 1.0]  GraphicAmbientColor=[0.15 0.15 0.15 1.0]  GraphicEmissiveColor=[0.0 0.0 0.0 1.0]  GraphicShininess=75  GraphicOpacity=0.2
  Mux1 : Mux  Inputs=5
  PS-Simulink Converter{1..4,16} (5 alike) : nesl_utility/PS-Simulink Converter  PhysicalDomain=network_engine_domain  SubClassName=ps_output  LeftPortType=input  RightPortType=output  PseudoPeriodic=off  Frequencies=[]  VectorFormat=inherit  Unit=inherit  AffineConversion=off
  Spatial Contact Force{7..10} (4 alike) : sm_lib/Forces and Torques/Spatial Contact Force  SenseContactBaseRotation=off  SenseContactBaseTranslation=off  CoefficientOfDynamicFriction=0.3  CoefficientOfStaticFriction=0.5  NormalDamping=1e3  NormalDampingUnits=N/(m/s)  SenseContactSignal=on  NormalStiffness=1e6  NormalStiffnessUnits=N/m  FrictionalCriticalVelocity=1e-3  FrictionalCriticalVelocityUnits=m/s  ZeroCrossDetectContactStartAndEnd=off  SenseContactFollowerRotation=off  SenseContactFollowerTranslation=off  FrictionType=SmoothStickSlip  SenseFrictionalForceMagnitude=off  SenseNormalForceMagnitude=off  NormalForceType=SmoothSpringDamper  SenseNormalVelocity=off  SensePenetrationDepth=off  SenseSeparationDistance=off  SenseTangentialVelocity=off  NormalTransitionRegionWidth=1e-4  NormalTransitionRegionWidthUnits=m
  Spatial Contact Force6 : sm_lib/Forces and Torques/Spatial Contact Force  SenseContactBaseRotation=off  SenseContactBaseTranslation=off  CoefficientOfDynamicFriction=0.3  CoefficientOfStaticFriction=0.5  NormalDamping=1e3  NormalDampingUnits=N/(m/s)  SenseContactSignal=on  NormalStiffness=1e6  NormalStiffnessUnits=N/m  FrictionalCriticalVelocity=1e-3  FrictionalCriticalVelocityUnits=m/s  ZeroCrossDetectContactStartAndEnd=on  SenseContactFollowerRotation=off  SenseContactFollowerTranslation=off  FrictionType=SmoothStickSlip  SenseFrictionalForceMagnitude=off  SenseNormalForceMagnitude=off  NormalForceType=SmoothSpringDamper  SenseNormalVelocity=off  SensePenetrationDepth=off  SenseSeparationDistance=off  SenseTangentialVelocity=off  NormalTransitionRegionWidth=1e-4  NormalTransitionRegionWidthUnits=m
  C1 : PMIOPort  Side=Left
  C2 : PMIOPort  Port=2  Side=Left
  C3 : PMIOPort  Port=3  Side=Left
  C4 : PMIOPort  Port=4  Side=Left
  C5 : PMIOPort  Port=5  Side=Left
  WR : PMIOPort  Port=6  Side=Right
  Col : Outport
  wires:
  PS-Simulink Converter4/1 -> Mux1/5  "5"
  PS-Simulink Converter3/1 -> Mux1/4  "4"
  PS-Simulink Converter16/1 -> Mux1/1  "1"
  PS-Simulink Converter1/1 -> Mux1/2  "2"
  PS-Simulink Converter2/1 -> Mux1/3  "3"
  Mux1/1 -> Col/1
  connections:
  Body/RConn1 -- WR/RConn1
  Body/LConn1 -- Spatial Contact Force10/LConn1 -- Spatial Contact Force9/LConn1 -- Spatial Contact Force8/LConn1 -- Spatial Contact Force7/LConn1 -- Spatial Contact Force6/LConn1
  Spatial Contact Force10/RConn1 -- C1/RConn1
  Spatial Contact Force8/RConn2 -- PS-Simulink Converter3/LConn1
  Spatial Contact Force7/RConn2 -- PS-Simulink Converter2/LConn1
  Spatial Contact Force9/RConn2 -- PS-Simulink Converter4/LConn1
  Spatial Contact Force6/RConn2 -- PS-Simulink Converter1/LConn1
  Spatial Contact Force10/RConn2 -- PS-Simulink Converter16/LConn1
  Spatial Contact Force6/RConn1 -- C2/RConn1
  Spatial Contact Force7/RConn1 -- C3/RConn1
  Spatial Contact Force8/RConn1 -- C4/RConn1
  Spatial Contact Force9/RConn1 -- C5/RConn1

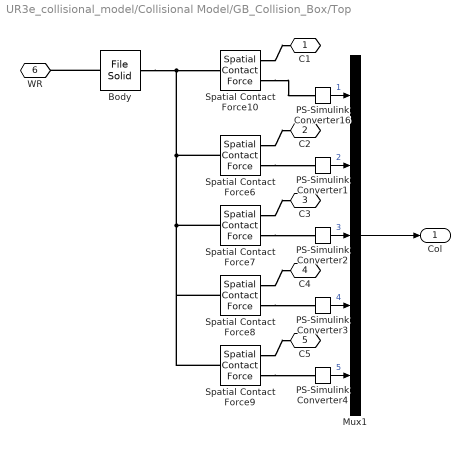
== system UR3e_collisional_model/Collisional Model/GB_Collision_Box/Top ==
  Body : sm_lib/Body Elements/File Solid  ExtGeomFileName=\UR3e_simscape_models\Glovebox_models\Top.stp  UnitType=FromFile  ExtGeomFileUnits=m  StepReaderType=HEX  ExportConvexHullGeometry=on  InertiaType=Custom  Mass=0  MassUnits=kg  CenterOfMass=[0 0 0]  CenterOfMassUnits=m  MomentsOfInertia=[1 1 1]  MomentsOfInertiaUnits=kg*m^2  ProductsOfInertia=[0 0 0]  ProductsOfInertiaUnits=kg*m^2  BasedOnType=DensityFromFile  Density=1000  DensityUnits=kg/m^3  DoExposeReferenceFrame=on  SerializedFrames=<Frames/>  GraphicType=FromGeometry  MarkerShape=Sphere  MarkerSize=10  GraphicVisPropType=SimpleVisualProperties  GraphicDiffuseColor=[1.0 1.0 1.0]  GraphicSpecularColor=[0.5 0.5 0.5 1.0]  GraphicAmbientColor=[0.15 0.15 0.15 1.0]  GraphicEmissiveColor=[0.0 0.0 0.0 1.0]  GraphicShininess=75  GraphicOpacity=0.2
  Mux1 : Mux  Inputs=5
  PS-Simulink Converter{1..4,16} (5 alike) : nesl_utility/PS-Simulink Converter  PhysicalDomain=network_engine_domain  SubClassName=ps_output  LeftPortType=input  RightPortType=output  PseudoPeriodic=off  Frequencies=[]  VectorFormat=inherit  Unit=inherit  AffineConversion=off
  Spatial Contact Force{7..10} (4 alike) : sm_lib/Forces and Torques/Spatial Contact Force  SenseContactBaseRotation=off  SenseContactBaseTranslation=off  CoefficientOfDynamicFriction=0.3  CoefficientOfStaticFriction=0.5  NormalDamping=1e3  NormalDampingUnits=N/(m/s)  SenseContactSignal=on  NormalStiffness=1e6  NormalStiffnessUnits=N/m  FrictionalCriticalVelocity=1e-3  FrictionalCriticalVelocityUnits=m/s  ZeroCrossDetectContactStartAndEnd=off  SenseContactFollowerRotation=off  SenseContactFollowerTranslation=off  FrictionType=SmoothStickSlip  SenseFrictionalForceMagnitude=off  SenseNormalForceMagnitude=off  NormalForceType=SmoothSpringDamper  SenseNormalVelocity=off  SensePenetrationDepth=off  SenseSeparationDistance=off  SenseTangentialVelocity=off  NormalTransitionRegionWidth=1e-4  NormalTransitionRegionWidthUnits=m
  Spatial Contact Force6 : sm_lib/Forces and Torques/Spatial Contact Force  SenseContactBaseRotation=off  SenseContactBaseTranslation=off  CoefficientOfDynamicFriction=0.3  CoefficientOfStaticFriction=0.5  NormalDamping=1e3  NormalDampingUnits=N/(m/s)  SenseContactSignal=on  NormalStiffness=1e6  NormalStiffnessUnits=N/m  FrictionalCriticalVelocity=1e-3  FrictionalCriticalVelocityUnits=m/s  ZeroCrossDetectContactStartAndEnd=on  SenseContactFollowerRotation=off  SenseContactFollowerTranslation=off  FrictionType=SmoothStickSlip  SenseFrictionalForceMagnitude=off  SenseNormalForceMagnitude=off  NormalForceType=SmoothSpringDamper  SenseNormalVelocity=off  SensePenetrationDepth=off  SenseSeparationDistance=off  SenseTangentialVelocity=off  NormalTransitionRegionWidth=1e-4  NormalTransitionRegionWidthUnits=m
  C1 : PMIOPort  Side=Left
  C2 : PMIOPort  Port=2  Side=Left
  C3 : PMIOPort  Port=3  Side=Left
  C4 : PMIOPort  Port=4  Side=Left
  C5 : PMIOPort  Port=5  Side=Left
  WR : PMIOPort  Port=6  Side=Right
  Col : Outport
  wires:
  PS-Simulink Converter4/1 -> Mux1/5  "5"
  PS-Simulink Converter3/1 -> Mux1/4  "4"
  PS-Simulink Converter16/1 -> Mux1/1  "1"
  PS-Simulink Converter1/1 -> Mux1/2  "2"
  PS-Simulink Converter2/1 -> Mux1/3  "3"
  Mux1/1 -> Col/1
  connections:
  Body/RConn1 -- WR/RConn1
  Body/LConn1 -- Spatial Contact Force10/LConn1 -- Spatial Contact Force9/LConn1 -- Spatial Contact Force8/LConn1 -- Spatial Contact Force7/LConn1 -- Spatial Contact Force6/LConn1
  Spatial Contact Force10/RConn1 -- C1/RConn1
  Spatial Contact Force8/RConn2 -- PS-Simulink Converter3/LConn1
  Spatial Contact Force7/RConn2 -- PS-Simulink Converter2/LConn1
  Spatial Contact Force9/RConn2 -- PS-Simulink Converter4/LConn1
  Spatial Contact Force6/RConn2 -- PS-Simulink Converter1/LConn1
  Spatial Contact Force10/RConn2 -- PS-Simulink Converter16/LConn1
  Spatial Contact Force6/RConn1 -- C2/RConn1
  Spatial Contact Force7/RConn1 -- C3/RConn1
  Spatial Contact Force8/RConn1 -- C4/RConn1
  Spatial Contact Force9/RConn1 -- C5/RConn1
